simulink model "penddemo"  (R2024a)
settings: Solver=FixedStepAuto  StartTime=0  StopTime=10  FixedStep=0.02  MaxStep=0.02  RelTol=1e-3  AbsTol=1e-6
model workspace (MAT data in the model file):
  input = 0
CloseFcn:
  | set(groot,'ShowHiddenHandles','on');
  | c = get(groot,'Children');
  | close(c);
  | clear c;
  | set(groot,'ShowHiddenHandles','off');
Description:
  | Inverted Pendulum with Animation
  | 
  | This example shows how to model an inverted pendulum.  The animation is created using MATLAB(R) Handle Graphics(R).  The animation block is a masked
  | S-function.  For more information, use the context menu to look under the Animation block's mask
  | and open the S-function for editing.
settings Model: PacingRate=0.500000  Creator=The MathWorks, Inc.  LastModifiedBy=ariellevy
settings SolverCC: AutoScaleAbsTol=off  AlgebraicLoopSolver=TrustRegion
settings DataIOCC: ExternalInput=[]  InitialState=[]  SaveFormat=Array  SaveOutput=off  SaveTime=off
settings OptimizationCC: BlockReduction=off  BooleanDataType=off  ReuseModelBlockBuffer=off  ExpressionDepthLimit=2147483647  InitFltsAndDblsToZero=on  LifeSpan=inf
settings DebuggingCC: SaveWithParameterizedLinksMsg=none  UnderspecifiedInitializationDetection=Classic  MergeDetectMultiDrivingBlocksExec=none  SignalResolutionControl=TryResolveAllWithWarning  MultiTaskDSMMsg=warning  MultiTaskCondExecSysMsg=none  SigSpecEnsureSampleTimeMsg=none  FcnCallInpInsideContextMsg=warning  UnconnectedInputMsg=warning  UnconnectedOutputMsg=warning  UnconnectedLineMsg=warning  StateNameClashWarn=warning  SubsystemReferenceDiagnosticForUnitTest=warning  SFUnexpectedBacktrackingDiag=warning  SFNoUnconditionalDefaultTransitionDiag=warning  SFExecutionAtInitializationDiag=none  ArithmeticOperatorsInVariantConditions=warning
settings HardwareCC: ProdBitPerPointer=32  ProdBitPerSizeT=32  ProdBitPerPtrDiffT=32  ProdLargestAtomicFloat=None  ProdIntDivRoundTo=Undefined  ProdEndianess=Unspecified  ProdWordSize=32  ProdHWDeviceType=32-bit Generic  TargetUnknown=on
settings ModelReferenceCC: EnableRefExpFcnMdlSchedulingChecks=on  PropagateSignalLabelsOutOfModel=off
settings SFSimCC: SimUseLocalCustomCode=off  CustomCodeUndefinedFunction=UseInterfaceOnly
settings RTWCC: RTWUseLocalCustomCode=off  GPUComputeCapability=3.5
settings CodeAppCC: StateflowObjectComments=on
settings GRTTargetCC: TargetFcnLib=ansi_tfl_tmw.mat  TargetLangStandard=C89/C90 (ANSI)  CombineOutputUpdateFcns=off  GRTInterface=on
settings ConfigComp: CovMetricSettings=dw  CovSaveCumulativeToWorkspaceVar=on  CovSaveSingleToWorkspaceVar=on  CovExternalEMLEnable=off

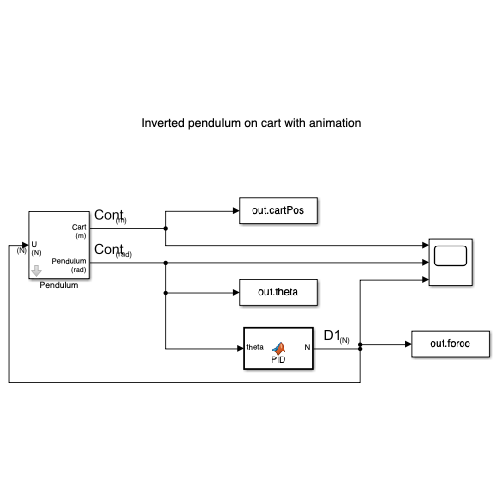
[thumbnail: Simulink's stored preview of the top-level diagram]
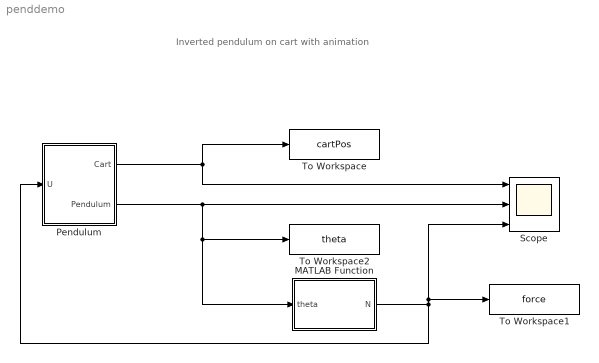
== system penddemo ==
  note: Inverted pendulum on cart with animation
  MATLAB Function : MATLAB Function  TreatAsAtomicUnit=on
  Pendulum : Subsystem  mask(Inverted Pendulum Dynamics){Mcart=0.455, m=0.21, l=0.61/2, g=9.8}
      mask prompts: Mcart "Mass of cart (kg):"; m "Mass of pendulum (kg):"; l "Distance to pendulum center of mass (m):"; g "Acceleration of gravity (m/s^2):"
      mask help: Masked subsystem containing nonlinear dynamics of inverted pendulum on a cart.
      mask Help: Nonlinear dynamics of inverted pendulum on cart.
  Scope : Scope  NumInputPorts=3
  To Workspace : ToWorkspace  VariableName=cartPos  SaveFormat=Timeseries  SampleTime=-1
  To Workspace1 : ToWorkspace  VariableName=force  SaveFormat=Timeseries  SampleTime=-1
  To Workspace2 : ToWorkspace  VariableName=theta  SaveFormat=Timeseries  SampleTime=-1
  wires:
  Pendulum/2(Pendulum) -> Scope/2, MATLAB Function/1(theta), To Workspace2/1
  Pendulum/1(Cart) -> Scope/1, To Workspace/1
  MATLAB Function/1(N) -> To Workspace1/1, Scope/3, Pendulum/1(U)

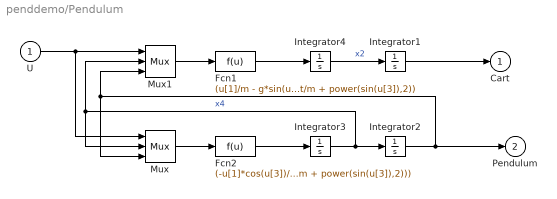
== system penddemo/Pendulum ==
  U : Inport  Unit=N
  Fcn1 : Fcn  Expr=(u[1]/m - g*sin(u[3])*cos(u[3]) + l*power(u[2],2)*sin(u[3]))/(Mcart/m + power(sin(u[3]),2))
  Fcn2 : Fcn  Expr=(-u[1]*cos(u[3])/m + (Mcart+m)*g*sin(u[3])/m - l*power(u[2],2)*sin(u[3])*cos(u[3]))/(l*(Mcart/m + power(sin(u[3]),2)))
  Integrator{1..4} (4 alike) : Integrator
  Mux : Mux  Inputs=3
  Mux1 : Mux  Inputs=3
  Cart : Outport  Unit=m  InitialOutput=0  VectorParamsAs1DForOutWhenUnconnected=off
  Pendulum : Outport  Port=2  Unit=rad  InitialOutput=0  VectorParamsAs1DForOutWhenUnconnected=off
  wires:
  Integrator1/1 -> Cart/1
  Fcn2/1 -> Integrator3/1
  Mux/1 -> Fcn2/1
  Mux1/1 -> Fcn1/1
  Fcn1/1 -> Integrator4/1
  Integrator4/1 -> Integrator1/1  "x2"
  U/1 -> Mux1/1, Mux/1
  Integrator3/1 -> Integrator2/1, Mux1/2, Mux/2  "x4"
  Integrator2/1 -> Pendulum/1, Mux1/3, Mux/3

== matlab function penddemo/MATLAB Function ==
  settings: updateMethod=DISCRETE
  data: N output; theta input
function N = PID(theta)

    % call extrinsic python function
    coder.extrinsic('py.PIDController.PIDRun');
    % Initialize offset angle
    persistent offset;
    if isempty(offset)
        % Offset the pendulum position on the first iteration
        offset = 0.1; % Adjust this value as needed
    else
        offset = 0; % No offset on subsequent iterations
    end
    % Add offset to theta
    theta = theta + offset;

    % Call Python function and return result
    N = coder.nullcopy(zeros(1,1)); % no clue why, but this is need.
    N = double(py.PIDController.PIDRun(theta, 0.02));
    disp(N);
end
